simulink model "EMPlanner_cs"  (R2020a)
settings: Solver=ode5  StartTime=0.0  StopTime=120  FixedStep=1/1000  RelTol=1e-3
PreLoadFcn:
  | mbxruntime.callbacks.PreLoadFcn(bdroot);
PostLoadFcn:
  | mbxruntime.callbacks.PostLoadFcn(bdroot);
InitFcn:
  | mbxruntime.callbacks.InitFcn(bdroot);
StartFcn:
  | mbxruntime.callbacks.StartFcn(bdroot);
StopFcn:
  | mbxruntime.callbacks.StopFcn(bdroot);
model workspace (MAT data in the model file):
  mbox_table : object (value not decoded)
  model_closed = 0
  sim_status = 0
undefined symbols (not defined in the file or in its folder): aubr, c_factor, cf, cr, DiscIntNeverNeededParam, global_path_x, global_path_y, KD_PID_distance, KD_PID_speed, KI_PID_distance, KI_PID_speed, KP_PID_distance, KP_PID_speed, la, lb, LQR_K1, LQR_K2, LQR_K3, LQR_K4, m, rack_displacement, right_wheel_ground, tablebr, vubr, vx_break_point, warningInitialVelocity, x0
libraries: PreScanSimulinkLibrary x33, simulink x19, simulink_extras x6, Solver_SF x1
(part 6 of 11)

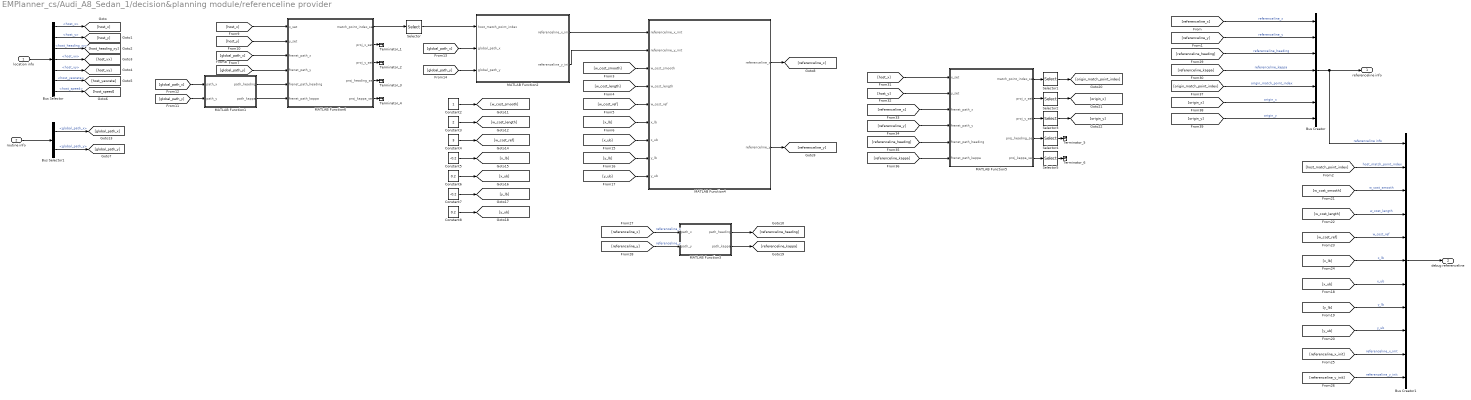
== system EMPlanner_cs/Audi_A8_Sedan_1/decision&planning module/referenceline provider ==
  location info : Inport
  routine info : Inport  Port=2
  Bus Creator : BusCreator  Inputs=7
  Bus Creator1 : BusCreator  Inputs=11
  Bus Selector : BusSelector  OutputSignals=host_x,host_y,host_heading_xy,host_vx,host_vy,host_yawrate,host_speed
  Bus Selector1 : BusSelector  OutputSignals=global_path_x,global_path_y
  Constant2 : Constant
  Constant3 : Constant  Value=2
  Constant4 : Constant  Value=3
  Constant5 : Constant  Value=-0.2
  Constant6 : Constant  Value=0.2
  Constant7 : Constant  Value=-0.2
  Constant8 : Constant  Value=0.2
  MATLAB Function1 : MATLAB Function  TreatAsAtomicUnit=on
  MATLAB Function2 : MATLAB Function  TreatAsAtomicUnit=on
  MATLAB Function3 : MATLAB Function  TreatAsAtomicUnit=on
  MATLAB Function4 : MATLAB Function  TreatAsAtomicUnit=on
  MATLAB Function5 : MATLAB Function  TreatAsAtomicUnit=on
  MATLAB Function6 : MATLAB Function  TreatAsAtomicUnit=on
  Selector{,1..5} (6 alike) : Selector  InputPortWidth=128  IndexOptions=Index vector (dialog)  Indices=1  OutputSizes=1
  Terminator_{1..6} (6 alike) : Terminator
  referenceline info : Outport
  debug referenceline : Outport  Port=2
  wires:
  [global_path_x] -> MATLAB Function2/2(global_path_x)
  [host_x] -> MATLAB Function6/1(x_set)
  MATLAB Function1/2(path_kappa) -> MATLAB Function6/6(frenet_path_kappa)
  MATLAB Function1/1(path_heading) -> MATLAB Function6/5(frenet_path_heading)
  [global_path_y] -> MATLAB Function6/4(frenet_path_y)
  [global_path_x] -> MATLAB Function6/3(frenet_path_x)
  [host_y] -> MATLAB Function6/2(y_set)
  [global_path_y] -> MATLAB Function1/2(path_y)
  [global_path_x] -> MATLAB Function1/1(path_x)
  Selector/1 -> MATLAB Function2/1(host_match_point_index)
  MATLAB Function6/1(match_point_index_set) -> Selector/1
  [global_path_y] -> MATLAB Function2/3(global_path_y)
  MATLAB Function2/1(referenceline_x_init) -> MATLAB Function4/1(referenceline_x_init)
  Bus Selector/5 -> [host_vy]  "<host_vy>"
  Bus Selector/1 -> [host_x]  "<host_x>"
  Bus Selector/2 -> [host_y]  "<host_y>"
  Bus Selector/3 -> [host_heading_xy]  "<host_heading_xy>"
  Bus Selector/4 -> [host_vx]  "<host_vx>"
  Bus Selector/7 -> [host_speed]  "<host_speed>"
  Bus Selector/6 -> [host_yawrate]  "<host_yawrate>"
  location info/1 -> Bus Selector/1
  Bus Selector1/2 -> [global_path_y]  "<global_path_y>"
  Bus Selector1/1 -> [global_path_x]  "<global_path_x>"
  routine info/1 -> Bus Selector1/1
  MATLAB Function4/1(referenceline_x) -> [referenceline_x]
  MATLAB Function4/2(referenceline_y) -> [referenceline_y]
  [referenceline_x] -> Bus Creator/1  "referenceline_x"
  [referenceline_y] -> Bus Creator/2  "referenceline_y"
  Bus Creator1/1 -> debug referenceline/1
  Bus Creator/1 -> Bus Creator1/1, referenceline info/1  "referenceline info"
  Constant2/1 -> [w_cost_smooth]
  Constant3/1 -> [w_cost_length]
  Constant8/1 -> [y_ub]
  Constant7/1 -> [y_lb]
  Constant6/1 -> [x_ub]
  Constant5/1 -> [x_lb]
  Constant4/1 -> [w_cost_ref]
  [w_cost_smooth] -> MATLAB Function4/3(w_cost_smooth)
  [w_cost_length] -> MATLAB Function4/4(w_cost_length)
  [w_cost_ref] -> MATLAB Function4/5(w_cost_ref)
  [x_lb] -> MATLAB Function4/6(x_lb)
  [x_ub] -> MATLAB Function4/7(x_ub)
  [y_lb] -> MATLAB Function4/8(y_lb)
  [y_ub] -> MATLAB Function4/9(y_ub)
  MATLAB Function2/2(referenceline_y_init) -> MATLAB Function4/2(referenceline_y_init)
  [w_cost_ref] -> Bus Creator1/5  "w_cost_ref"
  [x_lb] -> Bus Creator1/6  "x_lb"
  [w_cost_length] -> Bus Creator1/4  "w_cost_length"
  [x_ub] -> Bus Creator1/7  "x_ub"
  [w_cost_smooth] -> Bus Creator1/3  "w_cost_smooth"
  [y_lb] -> Bus Creator1/8  "y_lb"
  [host_match_point_index] -> Bus Creator1/2  "host_match_point_index"
  [y_ub] -> Bus Creator1/9  "y_ub"
  [referenceline_x_init] -> Bus Creator1/10  "referenceline_x_init"
  [referenceline_y_init] -> Bus Creator1/11  "referenceline_y_init"
  [referenceline_x] -> MATLAB Function3/1(path_x)  "referenceline_x"
  [referenceline_y] -> MATLAB Function3/2(path_y)  "referenceline_y"
  MATLAB Function3/1(path_heading) -> [referenceline_heading]
  MATLAB Function3/2(path_kappa) -> [referenceline_kappa]
  [referenceline_kappa] -> Bus Creator/4  "referenceline_kappa"
  [referenceline_heading] -> Bus Creator/3  "referenceline_heading"
  [host_x] -> MATLAB Function5/1(x_set)
  [host_y] -> MATLAB Function5/2(y_set)
  [referenceline_x] -> MATLAB Function5/3(frenet_path_x)
  [referenceline_y] -> MATLAB Function5/4(frenet_path_y)
  [referenceline_heading] -> MATLAB Function5/5(frenet_path_heading)
  [referenceline_kappa] -> MATLAB Function5/6(frenet_path_kappa)
  MATLAB Function5/1(match_point_index_set) -> Selector1/1
  MATLAB Function5/2(proj_x_set) -> Selector2/1
  MATLAB Function5/3(proj_y_set) -> Selector3/1
  MATLAB Function5/4(proj_heading_set) -> Selector4/1
  MATLAB Function5/5(proj_kappa_set) -> Selector5/1
  Selector1/1 -> [origin_match_point_index]
  Selector2/1 -> [origin_x]
  Selector3/1 -> [origin_y]
  [origin_match_point_index] -> Bus Creator/5  "origin_match_point_index"
  [origin_x] -> Bus Creator/6  "origin_x"
  [origin_y] -> Bus Creator/7  "origin_y"
  MATLAB Function6/2(proj_x_set) -> Terminator_1/1
  MATLAB Function6/3(proj_y_set) -> Terminator_2/1
  MATLAB Function6/4(proj_heading_set) -> Terminator_3/1
  MATLAB Function6/5(proj_kappa_set) -> Terminator_4/1
  Selector4/1 -> Terminator_5/1
  Selector5/1 -> Terminator_6/1

== system EMPlanner_cs/Audi_A8_Sedan_2/Dynamics_Simple/Chassis ==
  TransmissionTorque_[Nm] : Inport
  BrakePressure_[bar] : Inport  Port=2
  DeltaSteer_[deg] : Inport  Port=3
  Initial_Vx_[m s-1] : Inport  Port=4
  Abs : Abs
  Bicycle_model_[XYZ] : Subsystem
      mask Display: image(imread('Bicycle_model.png'));
  Constant3 : Constant  Value=[0 0]
  Constant4 : Constant  Value=[0 0]
  Degrees to Radians : simulink_extras/Transformations/Degrees to Radians
  FinalDriveRatio : Gain  Gain=p.Rfd  SaturateOnIntegerOverflow=on  OutDataTypeStr=Inherit: Same as input  ParamDataTypeStr=Inherit: Same as input
  "FinalDriveRatio " : Gain  Gain=p.Rfd  SaturateOnIntegerOverflow=on  OutDataTypeStr=Inherit: Same as input  ParamDataTypeStr=Inherit: Same as input
  FrontTyre : Subsystem
      mask Display: image(imread('Tyre.png'));
  Gain : Gain  Gain=2*pi/60
  MuxDynState : Subsystem
  Power Assisted Steering : Subsystem
  Product : Product  RndMeth=Zero
  RearTyre : Subsystem
      mask Display: image(imread('Tyre.png'));
  SteerRatio : Gain  Gain=1/p.SteerRatio
  Terminator4 : Terminator
  "[ms-1 --> rpm]" : Gain  Gain=60/(2*pi*p.Rw)  SaturateOnIntegerOverflow=on  OutDataTypeStr=Inherit: Same as input  ParamDataTypeStr=Inherit: Same as input
  to_kW : Gain  Gain=0.001
  State : Outport
  VehicleSpeed_[ms-1] : Outport  Port=2
  Vy_[ms-1] : Outport  Port=3
  ax_[ms-2] : Outport  Port=4
  ay_[ms-2] : Outport  Port=5
  PDrive_[kW] : Outport  Port=6
  TransmissionOut_[rpm] : Outport  Port=7
  wires:
  [vy] -> Vy_[ms-1]/1  "vy_[ms-1]"
  to_kW/1 -> PDrive_[kW]/1  "PDrive_[kW]"
  Gain/1 -> Product/1
  Bicycle_model_[XYZ]/10(ax_[ms-2]) -> ax_[ms-2]/1  "ax_[ms-2]"
  Product/1 -> to_kW/1
  [DT] -> Product/2
  Bicycle_model_[XYZ]/11(ay_[ms-2]) -> ay_[ms-2]/1  "ay_[ms-2]"
  Abs/1 -> Bicycle_model_[XYZ]/7(|vx|_[ms-1])
  Degrees to Radians/1 -> SteerRatio/1
  [vx] -> Abs/1
  SteerRatio/1 -> [DeltaWheel], Bicycle_model_[XYZ]/1(DeltaWheel_[rad])  "DeltaWheel_[rad]"
  TransmissionTorque_[Nm]/1 -> "FinalDriveRatio "/1  "DriveTorque_[Nm]"
  RearTyre/1(FyRear_[N]) -> Bicycle_model_[XYZ]/8(Fy_rear_[N])  "Fy_rear_[N]"
  FrontTyre/1(FyFront_[N]) -> Bicycle_model_[XYZ]/9(Fy_front_[N])  "Fy_front_[N]"
  Bicycle_model_[XYZ]/1(|vx|_[ms-1]1) -> [Absvx]  "|vx|_[ms-1]"
  Bicycle_model_[XYZ]/2(vy_[ms-1]) -> [vy], MuxDynState/2(vy [ms-1])  "Vy_[ms-1]"
  Bicycle_model_[XYZ]/4(RollAngle_[rad]) -> MuxDynState/4(R [rad]), [RollAngle]  "RollAngle_[rad]"
  Bicycle_model_[XYZ]/6(YawAngle_[rads-1]) -> [YawRate]  "YawRate_[rad s-1]"
  Bicycle_model_[XYZ]/7(Vx_[ms-1]) -> [vx]  "Vx_[ms-1]"
  [DeltaWheel] -> FrontTyre/1(DeltaWheel_[rad])
  [Absvx] -> FrontTyre/2(|vx|_[ms-1])
  [vy] -> FrontTyre/3(vy_[ms-1])
  [YawRate] -> FrontTyre/4(dYawAngle_[rads-1])
  [Absvx] -> RearTyre/1(|vx|_[ms-1])
  [vy] -> RearTyre/2(vy_[ms-1])
  [YawRate] -> RearTyre/3(dpsi_[rads-1])
  Bicycle_model_[XYZ]/3(vz_[ms-1]) -> MuxDynState/3(vz [ms-1])  "Vz_[ms-1]"
  Bicycle_model_[XYZ]/8(PitchAngle_[rad]) -> MuxDynState/5(P [rad])  "PitchAngle_[rad]"
  Bicycle_model_[XYZ]/9(YawAngle_[rad]) -> MuxDynState/6(Y [rad])  "YawAngle_[rad]"
  "[ms-1 --> rpm]"/1 -> Gain/1, FinalDriveRatio/1
  FinalDriveRatio/1 -> TransmissionOut_[rpm]/1  "TransmissionOut_[rpm]"
  [vx] -> "[ms-1 --> rpm]"/1, VehicleSpeed_[ms-1]/1, MuxDynState/1(vx [ms-1])  "vx_[ms-1]"
  [vx] -> Power Assisted Steering/1(Vx_[ms-1])
  DeltaSteer_[deg]/1 -> Power Assisted Steering/2(Delta_in_[deg])
  Power Assisted Steering/1(Delta_out_[deg]) -> Degrees to Radians/1
  [RollAngle] -> FrontTyre/5(RollAngle_[rad])
  [RollAngle] -> RearTyre/4(RollAngle_[rad])
  Constant3/1 -> Bicycle_model_[XYZ]/2(zFront_[m]_dzFront_[ms-1])  "zFront_[m]_dzFront_[m s-1]"
  Constant4/1 -> Bicycle_model_[XYZ]/3(zRear_[m]_dzRear_[ms-1])  "zRear_[m]_dzRear_[m s-1]"
  BrakePressure_[bar]/1 -> Bicycle_model_[XYZ]/4(BrakePressure_[bar])  "BrakePressure_[bar]"
  "FinalDriveRatio "/1 -> Bicycle_model_[XYZ]/5(DriveTorque_[Nm]), [DT]  "DriveTorque_[Nm]"
  Initial_Vx_[m s-1]/1 -> Bicycle_model_[XYZ]/6(v0_[ms-1])  "Initial_Vx_[m s-1]"
  Bicycle_model_[XYZ]/5(RollRate_[rads-1]) -> Terminator4/1  "RollRate_[rad s-1]"
  MuxDynState/1(State) -> State/1  "State"

== system EMPlanner_cs/Audi_A8_Sedan_2/Dynamics_Simple/Engine ==
  ImpellerTorque_[Nm] : Inport
  Throttle_[%] : Inport  Port=2
  Configurable Subsystem : Subsystem  BlockChoice=Rate Limiter  mask{ComputationMode=ComputationMode}
      mask prompts: ComputationMode "Compuation mode:"
      mask init:
      | SetComputationMode(gcb,ComputationMode);
      settings: AttributesFormatString=%<BlockChoice>  OpenFcn=BringToFront(gcb);  MemberBlocks=Discrete Rate Limiter,Rate Limiter
      settings: TemplateBlock=|
      | PreScanSimulinkLibrary/Configurable Subsystems/TransferFunction
      | Engine/Configurable
      | Subsystem
  Configurable Subsystem1 : Subsystem  BlockChoice=Integrator  mask{ComputationMode=ComputationMode}
      mask prompts: ComputationMode "Computation mode:"
      mask init:
      | SetComputationMode(gcb,ComputationMode);
      settings: AttributesFormatString=%<BlockChoice>  OpenFcn=BringToFront(gcb);  MemberBlocks=Discrete-Time Integrator,Integrator
      settings: TemplateBlock=|
      | PreScanSimulinkLibrary/Configurable Subsystems/integral with initial condition and limts
      | for engine/Configurable
      | Subsystem
  EngineTorque : Lookup2D  RowIndex=p.thvec  ColumnIndex=p.nevec  Table=p.emap  InputSameDT=on
  Gain : Gain  Gain=2*pi/60
  Product : Product  RndMeth=Zero
  Sum : Sum  Inputs=-+  InputSameDT=on  SaturateOnIntegerOverflow=on  OutDataTypeStr=Inherit: Same as first input
  engine + impeller inertia : Gain  Gain=1/p.Iei  SaturateOnIntegerOverflow=on  OutDataTypeStr=Inherit: Same as input  ParamDataTypeStr=Inherit: Same as input
  rad|sec2rpm : Gain  Gain=60/2/pi  SaturateOnIntegerOverflow=on  OutDataTypeStr=Inherit: Same as input  ParamDataTypeStr=Inherit: Same as input
  to_kW : Gain  Gain=0.001
  nEngine_[rpm] : Outport  InitialOutput=0
  PEngine_[kW] : Outport  Port=2  InitialOutput=0
  wires:
  rad|sec2rpm/1 -> nEngine_[rpm]/1, EngineTorque/2, Gain/1  "rpm"
  engine + impeller inertia/1 -> Configurable Subsystem1/1(In1)  "rads-2"
  EngineTorque/1 -> Sum/2, Product/2
  Sum/1 -> engine + impeller inertia/1
  Configurable Subsystem1/1(Out1) -> rad|sec2rpm/1  "rads-1"
  Throttle_[%]/1 -> Configurable Subsystem/1(In1)
  ImpellerTorque_[Nm]/1 -> Sum/1
  Configurable Subsystem/1(Out1) -> EngineTorque/1
  Product/1 -> to_kW/1
  Gain/1 -> Product/1
  to_kW/1 -> PEngine_[kW]/1

== system EMPlanner_cs/Audi_A8_Sedan_2/Dynamics_Simple/Gear: Auto Manual ==
  note: 0; Auto = on // Manual =off
      | 1; Auto = off // Manual =on
  Auto_Manual : Inport
  Manual_Gear : Inport  Port=2
  Auto_Gear : Inport  Port=3
  If : If  IfExpression=u1 == 0
  If Action Subsystem : Subsystem  TreatAsAtomicUnit=on
  If Action Subsystem1 : Subsystem  TreatAsAtomicUnit=on
  Merge : Merge
  Gear : Outport
  wires:
  If Action Subsystem/1(Out1) -> Merge/1
  Auto_Gear/1 -> If Action Subsystem/1(In1)
  If/1 -> If Action Subsystem/Action
  Merge/1 -> Gear/1
  If Action Subsystem1/1(Out1) -> Merge/2
  Manual_Gear/1 -> If Action Subsystem1/1(In1)
  If/2 -> If Action Subsystem1/Action
  Auto_Manual/1 -> If/1

== system EMPlanner_cs/Audi_A8_Sedan_2/Dynamics_Simple/ShiftLogic ==
  Throttle_[%] : Inport
  GearNr_[-] : Inport  Port=2
  Auto_GearShift : Inport  Port=3
  VehSpeed_[ms-1] : Inport  Port=4
  Add2 : Sum
  Data Type Conversion1 : DataTypeConversion  OutDataTypeStr=double
  Detect Increase1 : simulink/Logic and Bit Operations/Detect Increase  vinit=0.0  OutDataTypeStr=uint8
  Detect Increase : Subsystem
  Gear limitation : Saturate  UpperLimit=p.maxGear  LowerLimit=1
  Gear limitation while shifting : Saturate  UpperLimit=p.maxGear  LowerLimit=1
  GearNeutral : Constant  Value=0
  GearReverse : Constant  Value=-1
  "IC, gear = 1" : Memory  InitialCondition=1  InheritSampleTime=on
  If Action Neutral : Subsystem  TreatAsAtomicUnit=on
  If Action Normal : Subsystem  TreatAsAtomicUnit=on
  If Action Reverse : Subsystem  TreatAsAtomicUnit=on
  Memory : Memory  InheritSampleTime=on
  Merge : Merge  Inputs=3
  Relational Operator : RelationalOperator  OutDataTypeStr=boolean  RndMeth=Nearest
  Relational Operator1 : RelationalOperator  Operator=<=  OutDataTypeStr=boolean  RndMeth=Nearest
  Shift_Down time : Delay  DelayLength=p.ShiftDown_fac
  Shift_Up time : Delay  DelayLength=p.ShiftUp_fac
  Sum : Sum  Inputs=+-
  interp_down : Lookup2D  RowIndex=p.downth  ColumnIndex=[1:p.maxGear]  Table=p.downtab  LookUpMeth=Interpolation-Use End Values  InputSameDT=on
  interp_up : Lookup2D  RowIndex=p.upth  ColumnIndex=[1:p.maxGear]  Table=p.uptab  LookUpMeth=Interpolation-Use End Values  InputSameDT=on
  reverse/neutral/normal gear : If  IfExpression=u1 == 0  ElseIfExpressions=u1 < 0
  to_ms-1 : Gain  Gain=1/3.6
  "to_ms-1 " : Gain  Gain=1/3.6
  GearNr : Outport
  wires:
  Auto_GearShift/1 -> reverse/neutral/normal gear/1
  "IC, gear = 1"/1 -> If Action Normal/1(In1)
  Merge/1 -> GearNr/1
  If Action Reverse/1(Out1) -> Merge/2
  If Action Neutral/1(Out1) -> Merge/1
  If Action Normal/1(Out1) -> Merge/3
  reverse/neutral/normal gear/3 -> If Action Normal/Action
  reverse/neutral/normal gear/1 -> If Action Neutral/Action
  reverse/neutral/normal gear/2 -> If Action Reverse/Action
  GearReverse/1 -> If Action Reverse/1(In1)
  GearNeutral/1 -> If Action Neutral/1(In1)
  Shift_Down time/1 -> Sum/2
  Shift_Up time/1 -> Sum/1
  Detect Increase/1(Out1) -> Shift_Up time/1
  Data Type Conversion1/1 -> Shift_Down time/1
  Detect Increase1/1 -> Data Type Conversion1/1
  Sum/1 -> Add2/1
  Memory/1 -> Add2/2  "GearNr_[-]"
  Add2/1 -> Gear limitation while shifting/1
  Gear limitation while shifting/1 -> "IC, gear = 1"/1, Memory/1  "GearNr_[-]"
  Throttle_[%]/1 -> interp_down/1, interp_up/1
  Relational Operator/1 -> Detect Increase/2(In2)
  Relational Operator1/1 -> Detect Increase1/1
  interp_down/1 -> "to_ms-1 "/1
  VehSpeed_[ms-1]/1 -> Relational Operator/1, Relational Operator1/1
  interp_up/1 -> to_ms-1/1
  Gear limitation/1 -> interp_down/2, interp_up/2, Detect Increase/1(GearNr_[-])
  GearNr_[-]/1 -> Gear limitation/1
  to_ms-1/1 -> Relational Operator/2
  "to_ms-1 "/1 -> Relational Operator1/2

== system EMPlanner_cs/Audi_A8_Sedan_2/Dynamics_Simple/Transmission ==
  nEngine_[rpm] : Inport
  GearNr_[-] : Inport  Port=2
  n_TransmissionOut_[rpm] : Inport  Port=3
  Torque_Converter : Subsystem
      mask Display: image(imread('TorqueConverter.png'));
  Transmission_Ratio : Subsystem
  Viscous coupling : Lookup  InputValues=[-5:0.1:5]*p.m/4  Table=p.m/4*tanh([-5:0.1:5])
  ImpellerTorque_[Nm] : Outport  InitialOutput=0
  TransmissionTorque_[Nm] : Outport  Port=2  InitialOutput=0
  wires:
  Torque_Converter/2(TurbineTorque_[Nm]) -> Viscous coupling/1  "Converter_Torque_[Nm]"
  Transmission_Ratio/2(nTransmissionIn_[rpm]) -> Torque_Converter/2(nTransmission_[rpm])
  nEngine_[rpm]/1 -> Torque_Converter/1(nEngine_[rpm])
  GearNr_[-]/1 -> Transmission_Ratio/2(GearNr_[-]), Torque_Converter/3(Gear nr)
  n_TransmissionOut_[rpm]/1 -> Transmission_Ratio/3(nTransmissionOut_[rpm])
  Torque_Converter/1(ImpellerTorque_[Nm]) -> ImpellerTorque_[Nm]/1
  Transmission_Ratio/1(tTransmissionOut_[Nm]) -> TransmissionTorque_[Nm]/1
  Viscous coupling/1 -> Transmission_Ratio/1(tTransmissionIn_[Nm])

== system EMPlanner_cs/Audi_A8_Sedan_2/PathFollower_Preview_1/LateralController ==
  TrajOffset x,y,Y [m,m,deg] : Inport
  ActorOffset_Left(+) / Right(-) [m] : Inport  Port=2
  position x,y,Y [m,m,deg] : Inport  Port=3
  vx [m/s] : Inport  Port=4
  vy [m/s] : Inport  Port=5
  Yaw rate [deg/s] : Inport  Port=6
  CorneringStiffness_Tyres_Front [N/rad] : Inport  Port=7
  CorneringStiffness_Tyres_Rear [N/rad] : Inport  Port=8
  steering_ratio[-] : Inport  Port=9
  Avoid_0 : Saturate  UpperLimit=1000  LowerLimit=0.1
  CTRL REFERENCES : Subsystem
  Calculate delta steering error : Subsystem
      mask Display:
      | port_label('input', 1, 'v_x_vehicle [m/s]')
      | port_label('input', 2, 'v_x_vehicle_Min [m/s]')
      | port_label('input', 3, 't_Preview_LatCtrl [s]')
      | port_label('input', 4, 'v_y_vehicle [m/s]')
      | port_label('input', 5, 'yawrate_vehicle [rad/sec]')
      | port_label('input', 6, 'CorneringStiffness_Tyres_Front [N/rad]')
      | port_label('input', 7, 'CorneringStiffness_Tyres_Rear [N/rad]')
      | port_label('input', 8, 'm_vehicle_total [kg]')
      | port_label('input', 9, 'inertia_z_vehicle_total [kg m2]')
      | port_label('input', 10, 'e_Lat [m]')
      | port_label('input', 11, 'Distance_frontaxle_COG(+) [m]')
      | port_label('input', 12, 'wheel_base [m]')
      | port_label('output', 1, 'delta_steeringwheel [rad]')
  Const_t_Preview_LatCtrl[s] : Constant  Value=PreviewTime  SampleTime=CSSampleTime
  Const_v_x_Vehicle_Min[km|h] : Constant  Value=LowSpeedLimit  SampleTime=CSSampleTime
  Constant6 : Constant  SampleTime=CSSampleTime
  Demux : Demux  Outputs=3
  Demux1 : Demux  Outputs=3
  Distance_frontaxle_COG(+) [m] : Constant  Value=length_a  SampleTime=CSSampleTime
  Gain : Gain  Gain=1*pi/180
  Gain1 : Gain  Gain=1*pi/180
  Gain4 : Gain
  Memory : Memory  InheritSampleTime=on
  Memory1 : Memory  InheritSampleTime=on
  Memory2 : Memory  InheritSampleTime=on
  Mux : Mux  Inputs=3
  Mux1 : Mux  Inputs=3
  SteeringWheelAngle : Subsystem
  deg to rad : Gain  Gain=pi/180
  inertia_z_vehicle_total [kg m2] : Constant  Value=Jzz  SampleTime=CSSampleTime
  km|h to m|s : Gain  Gain=1/3.6
  m_vehicle_total_[kg] : Constant  Value=mass  SampleTime=CSSampleTime
  s_Preview_LatCtrl : Subsystem
  wheel_base [m] : Constant  Value=length_l  SampleTime=CSSampleTime
  Actor/Traj_distance [m] : Outport
  Actor/Traj_angle [deg] : Outport  Port=2
  delta_steerwheel [deg] : Outport  Port=3
  wires:
  km|h to m|s/1 -> Calculate delta steering error/2(In2), s_Preview_LatCtrl/2(v_x_Vehicle_Min[m|s])
  Gain/1 -> Mux/3
  Mux/1 -> CTRL REFERENCES/3(TrajOffset [m,m,rad])
  ActorOffset_Left(+) / Right(-) [m]/1 -> CTRL REFERENCES/4(ActorOffset_Left(+) / Right(-)_[m])
  Demux/1 -> Mux/1
  Demux/2 -> Mux/2
  Demux/3 -> Gain/1
  TrajOffset x,y,Y [m,m,deg]/1 -> Demux/1
  CTRL REFERENCES/2(Actor/Traj_angle [deg]) -> Actor/Traj_angle [deg]/1
  CTRL REFERENCES/1(Actor/Traj_distance [m]) -> Actor/Traj_distance [m]/1
  Calculate delta steering error/1(Out1) -> SteeringWheelAngle/1(Angle_Steering[rad])
  vx [m/s]/1 -> Memory1/1
  vy [m/s]/1 -> Memory2/1
  CorneringStiffness_Tyres_Front [N/rad]/1 -> Calculate delta steering error/6(In6)
  m_vehicle_total_[kg]/1 -> Calculate delta steering error/8(In8)
  inertia_z_vehicle_total [kg m2]/1 -> Calculate delta steering error/9(In9)
  steering_ratio[-]/1 -> SteeringWheelAngle/2(i_Steering[])
  SteeringWheelAngle/1(Angle_SteeringWheel[deg]) -> Gain4/1, Memory/1
  Memory/1 -> SteeringWheelAngle/3(Angle_SteeringWheel_Last[deg])
  Constant6/1 -> SteeringWheelAngle/4(LatCtrl1_Enable[0Off|1On])
  Avoid_0/1 -> Calculate delta steering error/3(In3), s_Preview_LatCtrl/3(t_Preview_LatCtrl[s])
  Const_v_x_Vehicle_Min[km|h]/1 -> km|h to m|s/1
  s_Preview_LatCtrl/1(s_Preview_LatCtrl[m]) -> CTRL REFERENCES/2(Position Preview Distance [m])
  Const_t_Preview_LatCtrl[s]/1 -> Avoid_0/1
  Gain4/1 -> delta_steerwheel [deg]/1
  Distance_frontaxle_COG(+) [m]/1 -> Calculate delta steering error/11(In11)
  CorneringStiffness_Tyres_Rear [N/rad]/1 -> Calculate delta steering error/7(In7)
  Yaw rate [deg/s]/1 -> deg to rad/1
  deg to rad/1 -> Calculate delta steering error/5(In5)
  Gain1/1 -> Mux1/3
  Demux1/1 -> Mux1/1
  Demux1/2 -> Mux1/2
  Demux1/3 -> Gain1/1
  position x,y,Y [m,m,deg]/1 -> Demux1/1
  Mux1/1 -> CTRL REFERENCES/1(Pos x,y,Y [m,m,rad])
  wheel_base [m]/1 -> Calculate delta steering error/12(In12)
  CTRL REFERENCES/3(e_Lat [m]) -> Calculate delta steering error/10(In10)
  Memory1/1 -> Calculate delta steering error/1(In1), s_Preview_LatCtrl/1(v_x_Vehicle[m|s])
  Memory2/1 -> Calculate delta steering error/4(In4)

== system EMPlanner_cs/Audi_A8_Sedan_2/PathFollower_Preview_1/LongitudinalController ==
  v_actual [m/s] : Inport
  Desired Velocity [m/s] : Inport  Port=2
  Initial Velocity [m/s] : Inport  Port=3
  Check_Initial_Velocity : Subsystem
  Demux : Demux  Outputs=3
  GearNormal : Constant
  "GearNormal " : Constant
  If Desired Velocity = 0 : Subsystem  TreatAsAtomicUnit=on
  If Desired Velocity ~= 0 : Subsystem  TreatAsAtomicUnit=on
  Memory External IC : Subsystem
  Merge : Merge
  Mux : Mux  Inputs=3
  Mux2 : Mux  Inputs=3
  Sum4 : Sum  Inputs=|+-
  if : If  IfExpression=u1 == 0  SampleTime=CSSampleTime
  throttle [%] : Outport
  brake pressure [bar] : Outport  Port=2
  v0 [m/s] : Outport  Port=3
  Auto_GearShift : Outport  Port=4
  wires:
  v_actual [m/s]/1 -> Check_Initial_Velocity/1(" v_actual_[m|s]"), Memory External IC/1(u)
  Memory External IC/1(y) -> Sum4/2
  Sum4/1 -> If Desired Velocity ~= 0/2(Desired Velocity [m/s])
  Desired Velocity [m/s]/1 -> if/1, Sum4/1
  Initial Velocity [m/s]/1 -> Check_Initial_Velocity/2(Initial_Velocity_[m|s]), Memory External IC/2(IC), v0 [m/s]/1
  GearNormal/1 -> If Desired Velocity = 0/1(In1)
  Merge/1 -> Demux/1
  If Desired Velocity = 0/1(throttle [%]) -> Mux/1
  If Desired Velocity = 0/2(brake pressure [bar]) -> Mux/2
  Mux2/1 -> Merge/2
  Mux/1 -> Merge/1
  Demux/1 -> throttle [%]/1
  Demux/2 -> brake pressure [bar]/1
  Demux/3 -> Auto_GearShift/1
  "GearNormal "/1 -> If Desired Velocity ~= 0/1(In1)
  If Desired Velocity = 0/3(Auto_GearShift) -> Mux/3
  if/2 -> If Desired Velocity ~= 0/Action
  if/1 -> If Desired Velocity = 0/Action
  If Desired Velocity ~= 0/1(throttle [%]) -> Mux2/1
  If Desired Velocity ~= 0/2(brake pressure [bar]) -> Mux2/2
  If Desired Velocity ~= 0/3(Auto_GearShift) -> Mux2/3

== system EMPlanner_cs/Audi_A8_Sedan_2/SELF_Demux/compas converter ==
  rotz [rad] : Inport
  cart2compas : Subsystem
  rad2deg : Gain  Gain=180/pi
  heading [deg] : Outport
  wires:
  rad2deg/1 -> cart2compas/1(Angle [deg])
  rotz [rad]/1 -> rad2deg/1
  cart2compas/1(heading [deg]) -> heading [deg]/1

== system EMPlanner_cs/Audi_A8_Sedan_2/Trajectories/Traj2State1 ==
  Traj Org : Inport
  Offset : Inport  Port=2
  Add2 : Sum
  ApplyRotation : PreScanSimulinkLibrary/ApplyRotation  SystemSampleTime=-1  Latency=0  AutoFrameSizeCalculation=off
  ApplyRotation1 : PreScanSimulinkLibrary/ApplyRotation  SystemSampleTime=-1  Latency=0  AutoFrameSizeCalculation=off
  ApplyRotation2 : PreScanSimulinkLibrary/ApplyRotation  SystemSampleTime=-1  Latency=0  AutoFrameSizeCalculation=off
  Constant : Constant  Value=zeros(12,1)
  Mux : Mux  Inputs=6
  Mux1 : Mux  Inputs=2
  Mux{2,4..9} (7 alike) : Mux  Inputs=3
  Mux3 : Mux  Inputs=2
  Selector : Selector  InputPortWidth=6  IndexOptions=Index vector (dialog)  Indices=[4 5 6]  OutputSizes=1
  Selector1 : Selector  InputPortWidth=21  IndexOptions=Index vector (dialog)  Indices=[5]  OutputSizes=1
  Selector10 : Selector  InputPortWidth=21  IndexOptions=Index vector (dialog)  Indices=[2]  OutputSizes=1
  Selector11 : Selector  InputPortWidth=21  IndexOptions=Index vector (dialog)  Indices=[3]  OutputSizes=1
  Selector12 : Selector  InputPortWidth=21  IndexOptions=Index vector (dialog)  Indices=[1]  OutputSizes=1
  Selector13 : Selector  InputPortWidth=21  IndexOptions=Index vector (dialog)  Indices=[8]  OutputSizes=1
  Selector14 : Selector  InputPortWidth=21  IndexOptions=Index vector (dialog)  Indices=[9]  OutputSizes=1
  Selector15 : Selector  InputPortWidth=21  IndexOptions=Index vector (dialog)  Indices=[7]  OutputSizes=1
  Selector16 : Selector  InputPortWidth=21  IndexOptions=Index vector (dialog)  Indices=[14]  OutputSizes=1
  Selector17 : Selector  InputPortWidth=21  IndexOptions=Index vector (dialog)  Indices=[15]  OutputSizes=1
  Selector18 : Selector  InputPortWidth=21  IndexOptions=Index vector (dialog)  Indices=[13]  OutputSizes=1
  Selector19 : Selector  InputPortWidth=21  IndexOptions=Index vector (dialog)  Indices=[20]  OutputSizes=1
  Selector2 : Selector  InputPortWidth=21  IndexOptions=Index vector (dialog)  Indices=[6]  OutputSizes=1
  Selector20 : Selector  InputPortWidth=21  IndexOptions=Index vector (dialog)  Indices=[21]  OutputSizes=1
  Selector21 : Selector  InputPortWidth=21  IndexOptions=Index vector (dialog)  Indices=[19]  OutputSizes=1
  Selector3 : Selector  InputPortWidth=21  IndexOptions=Index vector (dialog)  Indices=[12]  OutputSizes=1
  Selector4 : Selector  InputPortWidth=21  IndexOptions=Index vector (dialog)  Indices=[17]  OutputSizes=1
  Selector5 : Selector  InputPortWidth=21  IndexOptions=Index vector (dialog)  Indices=[18]  OutputSizes=1
  Selector6 : Selector  InputPortWidth=21  IndexOptions=Index vector (dialog)  Indices=[16]  OutputSizes=1
  Selector7 : Selector  InputPortWidth=21  IndexOptions=Index vector (dialog)  Indices=[11]  OutputSizes=1
  Selector8 : Selector  InputPortWidth=21  IndexOptions=Index vector (dialog)  Indices=[10]  OutputSizes=1
  Selector9 : Selector  InputPortWidth=21  IndexOptions=Index vector (dialog)  Indices=[4]  OutputSizes=1
  Traj2State2 : Subsystem
  state : Outport
  wires:
  Mux9/1 -> ApplyRotation2/2, ApplyRotation1/2, ApplyRotation/2
  Selector20/1 -> Mux9/3
  Selector19/1 -> Mux9/2
  Selector21/1 -> Mux9/1
  Selector5/1 -> Mux8/3
  Selector4/1 -> Mux8/2
  Selector6/1 -> Mux8/1
  Mux8/1 -> Mux/6
  Mux6/1 -> ApplyRotation2/1
  Mux7/1 -> Mux/4
  ApplyRotation2/1 -> Mux/5
  Selector3/1 -> Mux7/3
  Selector7/1 -> Mux7/2
  Selector8/1 -> Mux7/1
  Mux4/1 -> Mux/2
  Mux5/1 -> ApplyRotation1/1
  ApplyRotation1/1 -> Mux/3
  Mux2/1 -> ApplyRotation/1
  ApplyRotation/1 -> Mux/1
  Selector2/1 -> Mux4/3
  Selector1/1 -> Mux4/2
  Selector9/1 -> Mux4/1
  Selector17/1 -> Mux6/3
  Selector16/1 -> Mux6/2
  Selector18/1 -> Mux6/1
  Selector14/1 -> Mux5/3
  Selector13/1 -> Mux5/2
  Selector15/1 -> Mux5/1
  Selector11/1 -> Mux2/3
  Selector10/1 -> Mux2/2
  Selector12/1 -> Mux2/1
  Mux3/1 -> Selector8/1, Selector7/1, Selector3/1, Selector18/1, Selector16/1, Selector17/1, Selector6/1, Selector20/1, Selector19/1, Selector21/1, Selector5/1, Selector4/1, Selector14/1, Selector13/1, Selector15/1, Selector2/1, Selector1/1, Selector9/1, Selector12/1, Selector10/1, Selector11/1
  Mux1/1 -> Add2/2
  Constant/1 -> Mux1/2
  Add2/1 -> Traj2State2/1(traj)
  Selector/1 -> Mux3/2
  Traj Org/1 -> Mux3/1
  Offset/1 -> Mux1/1, Selector/1
  Mux/1 -> Add2/1
  Traj2State2/1(state) -> state/1

== system EMPlanner_cs/Audi_A8_Sedan_2/Trajectories/TrajCoGOffset ==
  State In : Inport
  Add : Sum  Inputs=+-+
  Add1 : Sum
  ApplyRotation : PreScanSimulinkLibrary/ApplyRotation  SystemSampleTime=-1  Latency=0  AutoFrameSizeCalculation=off
  ApplyRotation1 : PreScanSimulinkLibrary/ApplyRotation  SystemSampleTime=-1  Latency=0  AutoFrameSizeCalculation=off
  CoG Offset : Constant  Value=[0 0 CoGOffsetZ]
  Degrees to Radians : simulink_extras/Transformations/Degrees to Radians
  Demux1 : Demux  Outputs=[3 3 3]
  Mux : Mux  Inputs=[3 3 3]
  Orientation : Constant  Value=[InitRoll InitPitch 0]
  State Out : Outport
  wires:
  State In/1 -> Demux1/1
  Demux1/1 -> Add/1
  Add/1 -> Mux/1
  Demux1/3 -> Mux/3, Add1/2
  Mux/1 -> State Out/1
  Demux1/2 -> Mux/2
  Orientation/1 -> Degrees to Radians/1
  ApplyRotation/1 -> Add/3
  ApplyRotation1/1 -> Add/2
  Add1/1 -> ApplyRotation/2
  CoG Offset/1 -> ApplyRotation1/1, ApplyRotation/1
  Degrees to Radians/1 -> Add1/1, ApplyRotation1/2

== system EMPlanner_cs/Audi_A8_Sedan_2/Trajectories/Trajectory_1 ==
  From Workspace : FromWorkspace  VariableName=trajectory  SampleTime=TimeStep  ZeroCross=off  OutputAfterFinalValue=Holding final value
  From Workspace1 : FromWorkspace  VariableName=trajectory  SampleTime=TimeStep  ZeroCross=off  OutputAfterFinalValue=Setting to zero
  Mux : Mux  Inputs=2
  Selector1 : Selector  InputPortWidth=24  IndexOptions=Index vector (dialog)  Indices=[7:18]  OutputSizes=1
  Selector9 : Selector  InputPortWidth=24  IndexOptions=Index vector (dialog)  Indices=[1:6]  OutputSizes=1
  trajectory : Outport
  wires:
  From Workspace/1 -> Selector9/1
  From Workspace1/1 -> Selector1/1
  Mux/1 -> trajectory/1
  Selector9/1 -> Mux/1
  Selector1/1 -> Mux/2

== system EMPlanner_cs/Box_1/Dynamics_Empty/MuxState ==
  note: mode: Dynamics
  note: mode: Positioning
  note: mode: Dynamics
      | VelVEHICLE
      | wrt VEH
  note: AnglesVEHICLE
      | wrtGLOB
  note: For state mode 'Dynamic' positions
      | are not taken into account, as they
      | are computed by integrating velocity.
      | Click annotation for Help.
  x [m] : Inport  SampleTime=TimeStep
  y [m] : Inport  Port=2  SampleTime=TimeStep
  z [m] : Inport  Port=3  SampleTime=TimeStep
  dx [m/s] : Inport  Port=4  SampleTime=TimeStep
  dy [m/s] : Inport  Port=5  SampleTime=TimeStep
  dz [m/s] : Inport  Port=6  SampleTime=TimeStep
  R [rad] : Inport  Port=7  SampleTime=TimeStep
  P [rad] : Inport  Port=8  SampleTime=TimeStep
  Y [rad] : Inport  Port=9  SampleTime=TimeStep
  Constant : Constant  DisableCoverage=on  Value=positioningmode
  Discrete-Time Integrator : DiscreteIntegrator  SampleTime=TimeStep  ICPrevOutput=DiscIntNeverNeededParam  ICPrevScaledInput=DiscIntNeverNeededParam
  Ground : Ground
  Ground1 : Ground
  Mux1 : Mux  Inputs=[3 3]
  Mux2 : Mux  Inputs=3
  Mux3 : Mux  Inputs=3
  Mux4 : Mux  Inputs=3
  Mux5 : Mux  Inputs=[3 3]
  Mux6 : Mux  Inputs=[6 3]
  Switch : Switch  Threshold=0.5
  Transformation_BODY2GLOBAL : PreScanSimulinkLibrary/Simple_Vehicle_Dynamics/Chassis/MuxDynState/Transformation_BODY2GLOBAL  SystemSampleTime=-1  Latency=0  AutoFrameSizeCalculation=off
  mux3 : Mux  Inputs=3
  state : Outport
  wires:
  Constant/1 -> Switch/2
  Mux6/1 -> state/1
  Mux4/1 -> Mux1/1
  Mux5/1 -> Switch/3
  Mux1/1 -> Switch/1
  Switch/1 -> Mux6/1  "PosVeh wrt  GLOB"
  P [rad]/1 -> Mux3/2
  R [rad]/1 -> Mux3/1
  dz [m/s]/1 -> Mux2/3
  dy [m/s]/1 -> Mux2/2
  dx [m/s]/1 -> Mux2/1
  z [m]/1 -> Mux4/3
  y [m]/1 -> Mux4/2
  x [m]/1 -> Mux4/1
  Ground1/1 -> mux3/2  "pitch"
  Y [rad]/1 -> mux3/3, Mux3/3  "yaw"
  Mux3/1 -> Mux6/2
  Transformation_BODY2GLOBAL/1 -> Discrete-Time Integrator/1, Mux5/2  "VelVEH wrt  GLOB"
  mux3/1 -> Transformation_BODY2GLOBAL/2
  Ground/1 -> mux3/1  "roll"
  Mux2/1 -> Mux1/2, Transformation_BODY2GLOBAL/1
  Discrete-Time Integrator/1 -> Mux5/1  "PosVEH wrt  GLOB"

== system EMPlanner_cs/Box_1/SELF_Demux/compas converter ==
  rotz [rad] : Inport
  cart2compas : Subsystem
  rad2deg : Gain  Gain=180/pi
  heading [deg] : Outport
  wires:
  rad2deg/1 -> cart2compas/1(Angle [deg])
  rotz [rad]/1 -> rad2deg/1
  cart2compas/1(heading [deg]) -> heading [deg]/1

== system EMPlanner_cs/Box_10/Dynamics_Empty/MuxState ==
  note: mode: Dynamics
  note: mode: Positioning
  note: mode: Dynamics
      | VelVEHICLE
      | wrt VEH
  note: AnglesVEHICLE
      | wrtGLOB
  note: For state mode 'Dynamic' positions
      | are not taken into account, as they
      | are computed by integrating velocity.
      | Click annotation for Help.
  x [m] : Inport  SampleTime=TimeStep
  y [m] : Inport  Port=2  SampleTime=TimeStep
  z [m] : Inport  Port=3  SampleTime=TimeStep
  dx [m/s] : Inport  Port=4  SampleTime=TimeStep
  dy [m/s] : Inport  Port=5  SampleTime=TimeStep
  dz [m/s] : Inport  Port=6  SampleTime=TimeStep
  R [rad] : Inport  Port=7  SampleTime=TimeStep
  P [rad] : Inport  Port=8  SampleTime=TimeStep
  Y [rad] : Inport  Port=9  SampleTime=TimeStep
  Constant : Constant  DisableCoverage=on  Value=positioningmode
  Discrete-Time Integrator : DiscreteIntegrator  SampleTime=TimeStep  ICPrevOutput=DiscIntNeverNeededParam  ICPrevScaledInput=DiscIntNeverNeededParam
  Ground : Ground
  Ground1 : Ground
  Mux1 : Mux  Inputs=[3 3]
  Mux2 : Mux  Inputs=3
  Mux3 : Mux  Inputs=3
  Mux4 : Mux  Inputs=3
  Mux5 : Mux  Inputs=[3 3]
  Mux6 : Mux  Inputs=[6 3]
  Switch : Switch  Threshold=0.5
  Transformation_BODY2GLOBAL : PreScanSimulinkLibrary/Simple_Vehicle_Dynamics/Chassis/MuxDynState/Transformation_BODY2GLOBAL  SystemSampleTime=-1  Latency=0  AutoFrameSizeCalculation=off
  mux3 : Mux  Inputs=3
  state : Outport
  wires:
  Constant/1 -> Switch/2
  Mux6/1 -> state/1
  Mux4/1 -> Mux1/1
  Mux5/1 -> Switch/3
  Mux1/1 -> Switch/1
  Switch/1 -> Mux6/1  "PosVeh wrt  GLOB"
  P [rad]/1 -> Mux3/2
  R [rad]/1 -> Mux3/1
  dz [m/s]/1 -> Mux2/3
  dy [m/s]/1 -> Mux2/2
  dx [m/s]/1 -> Mux2/1
  z [m]/1 -> Mux4/3
  y [m]/1 -> Mux4/2
  x [m]/1 -> Mux4/1
  Ground1/1 -> mux3/2  "pitch"
  Y [rad]/1 -> mux3/3, Mux3/3  "yaw"
  Mux3/1 -> Mux6/2
  Transformation_BODY2GLOBAL/1 -> Discrete-Time Integrator/1, Mux5/2  "VelVEH wrt  GLOB"
  mux3/1 -> Transformation_BODY2GLOBAL/2
  Ground/1 -> mux3/1  "roll"
  Mux2/1 -> Mux1/2, Transformation_BODY2GLOBAL/1
  Discrete-Time Integrator/1 -> Mux5/1  "PosVEH wrt  GLOB"

== system EMPlanner_cs/Box_10/SELF_Demux/compas converter ==
  rotz [rad] : Inport
  cart2compas : Subsystem
  rad2deg : Gain  Gain=180/pi
  heading [deg] : Outport
  wires:
  rad2deg/1 -> cart2compas/1(Angle [deg])
  rotz [rad]/1 -> rad2deg/1
  cart2compas/1(heading [deg]) -> heading [deg]/1

== system EMPlanner_cs/Box_11/Dynamics_Empty/MuxState ==
  note: mode: Dynamics
  note: mode: Positioning
  note: mode: Dynamics
      | VelVEHICLE
      | wrt VEH
  note: AnglesVEHICLE
      | wrtGLOB
  note: For state mode 'Dynamic' positions
      | are not taken into account, as they
      | are computed by integrating velocity.
      | Click annotation for Help.
  x [m] : Inport  SampleTime=TimeStep
  y [m] : Inport  Port=2  SampleTime=TimeStep
  z [m] : Inport  Port=3  SampleTime=TimeStep
  dx [m/s] : Inport  Port=4  SampleTime=TimeStep
  dy [m/s] : Inport  Port=5  SampleTime=TimeStep
  dz [m/s] : Inport  Port=6  SampleTime=TimeStep
  R [rad] : Inport  Port=7  SampleTime=TimeStep
  P [rad] : Inport  Port=8  SampleTime=TimeStep
  Y [rad] : Inport  Port=9  SampleTime=TimeStep
  Constant : Constant  DisableCoverage=on  Value=positioningmode
  Discrete-Time Integrator : DiscreteIntegrator  SampleTime=TimeStep  ICPrevOutput=DiscIntNeverNeededParam  ICPrevScaledInput=DiscIntNeverNeededParam
  Ground : Ground
  Ground1 : Ground
  Mux1 : Mux  Inputs=[3 3]
  Mux2 : Mux  Inputs=3
  Mux3 : Mux  Inputs=3
  Mux4 : Mux  Inputs=3
  Mux5 : Mux  Inputs=[3 3]
  Mux6 : Mux  Inputs=[6 3]
  Switch : Switch  Threshold=0.5
  Transformation_BODY2GLOBAL : PreScanSimulinkLibrary/Simple_Vehicle_Dynamics/Chassis/MuxDynState/Transformation_BODY2GLOBAL  SystemSampleTime=-1  Latency=0  AutoFrameSizeCalculation=off
  mux3 : Mux  Inputs=3
  state : Outport
  wires:
  Constant/1 -> Switch/2
  Mux6/1 -> state/1
  Mux4/1 -> Mux1/1
  Mux5/1 -> Switch/3
  Mux1/1 -> Switch/1
  Switch/1 -> Mux6/1  "PosVeh wrt  GLOB"
  P [rad]/1 -> Mux3/2
  R [rad]/1 -> Mux3/1
  dz [m/s]/1 -> Mux2/3
  dy [m/s]/1 -> Mux2/2
  dx [m/s]/1 -> Mux2/1
  z [m]/1 -> Mux4/3
  y [m]/1 -> Mux4/2
  x [m]/1 -> Mux4/1
  Ground1/1 -> mux3/2  "pitch"
  Y [rad]/1 -> mux3/3, Mux3/3  "yaw"
  Mux3/1 -> Mux6/2
  Transformation_BODY2GLOBAL/1 -> Discrete-Time Integrator/1, Mux5/2  "VelVEH wrt  GLOB"
  mux3/1 -> Transformation_BODY2GLOBAL/2
  Ground/1 -> mux3/1  "roll"
  Mux2/1 -> Mux1/2, Transformation_BODY2GLOBAL/1
  Discrete-Time Integrator/1 -> Mux5/1  "PosVEH wrt  GLOB"

== system EMPlanner_cs/Box_11/SELF_Demux/compas converter ==
  rotz [rad] : Inport
  cart2compas : Subsystem
  rad2deg : Gain  Gain=180/pi
  heading [deg] : Outport
  wires:
  rad2deg/1 -> cart2compas/1(Angle [deg])
  rotz [rad]/1 -> rad2deg/1
  cart2compas/1(heading [deg]) -> heading [deg]/1

== system EMPlanner_cs/Box_12/Dynamics_Empty/MuxState ==
  note: mode: Dynamics
  note: mode: Positioning
  note: mode: Dynamics
      | VelVEHICLE
      | wrt VEH
  note: AnglesVEHICLE
      | wrtGLOB
  note: For state mode 'Dynamic' positions
      | are not taken into account, as they
      | are computed by integrating velocity.
      | Click annotation for Help.
  x [m] : Inport  SampleTime=TimeStep
  y [m] : Inport  Port=2  SampleTime=TimeStep
  z [m] : Inport  Port=3  SampleTime=TimeStep
  dx [m/s] : Inport  Port=4  SampleTime=TimeStep
  dy [m/s] : Inport  Port=5  SampleTime=TimeStep
  dz [m/s] : Inport  Port=6  SampleTime=TimeStep
  R [rad] : Inport  Port=7  SampleTime=TimeStep
  P [rad] : Inport  Port=8  SampleTime=TimeStep
  Y [rad] : Inport  Port=9  SampleTime=TimeStep
  Constant : Constant  DisableCoverage=on  Value=positioningmode
  Discrete-Time Integrator : DiscreteIntegrator  SampleTime=TimeStep  ICPrevOutput=DiscIntNeverNeededParam  ICPrevScaledInput=DiscIntNeverNeededParam
  Ground : Ground
  Ground1 : Ground
  Mux1 : Mux  Inputs=[3 3]
  Mux2 : Mux  Inputs=3
  Mux3 : Mux  Inputs=3
  Mux4 : Mux  Inputs=3
  Mux5 : Mux  Inputs=[3 3]
  Mux6 : Mux  Inputs=[6 3]
  Switch : Switch  Threshold=0.5
  Transformation_BODY2GLOBAL : PreScanSimulinkLibrary/Simple_Vehicle_Dynamics/Chassis/MuxDynState/Transformation_BODY2GLOBAL  SystemSampleTime=-1  Latency=0  AutoFrameSizeCalculation=off
  mux3 : Mux  Inputs=3
  state : Outport
  wires:
  Constant/1 -> Switch/2
  Mux6/1 -> state/1
  Mux4/1 -> Mux1/1
  Mux5/1 -> Switch/3
  Mux1/1 -> Switch/1
  Switch/1 -> Mux6/1  "PosVeh wrt  GLOB"
  P [rad]/1 -> Mux3/2
  R [rad]/1 -> Mux3/1
  dz [m/s]/1 -> Mux2/3
  dy [m/s]/1 -> Mux2/2
  dx [m/s]/1 -> Mux2/1
  z [m]/1 -> Mux4/3
  y [m]/1 -> Mux4/2
  x [m]/1 -> Mux4/1
  Ground1/1 -> mux3/2  "pitch"
  Y [rad]/1 -> mux3/3, Mux3/3  "yaw"
  Mux3/1 -> Mux6/2
  Transformation_BODY2GLOBAL/1 -> Discrete-Time Integrator/1, Mux5/2  "VelVEH wrt  GLOB"
  mux3/1 -> Transformation_BODY2GLOBAL/2
  Ground/1 -> mux3/1  "roll"
  Mux2/1 -> Mux1/2, Transformation_BODY2GLOBAL/1
  Discrete-Time Integrator/1 -> Mux5/1  "PosVEH wrt  GLOB"

== system EMPlanner_cs/Box_12/SELF_Demux/compas converter ==
  rotz [rad] : Inport
  cart2compas : Subsystem
  rad2deg : Gain  Gain=180/pi
  heading [deg] : Outport
  wires:
  rad2deg/1 -> cart2compas/1(Angle [deg])
  rotz [rad]/1 -> rad2deg/1
  cart2compas/1(heading [deg]) -> heading [deg]/1

== system EMPlanner_cs/Box_2/Dynamics_Empty/MuxState ==
  note: mode: Dynamics
  note: mode: Positioning
  note: mode: Dynamics
      | VelVEHICLE
      | wrt VEH
  note: AnglesVEHICLE
      | wrtGLOB
  note: For state mode 'Dynamic' positions
      | are not taken into account, as they
      | are computed by integrating velocity.
      | Click annotation for Help.
  x [m] : Inport  SampleTime=TimeStep
  y [m] : Inport  Port=2  SampleTime=TimeStep
  z [m] : Inport  Port=3  SampleTime=TimeStep
  dx [m/s] : Inport  Port=4  SampleTime=TimeStep
  dy [m/s] : Inport  Port=5  SampleTime=TimeStep
  dz [m/s] : Inport  Port=6  SampleTime=TimeStep
  R [rad] : Inport  Port=7  SampleTime=TimeStep
  P [rad] : Inport  Port=8  SampleTime=TimeStep
  Y [rad] : Inport  Port=9  SampleTime=TimeStep
  Constant : Constant  DisableCoverage=on  Value=positioningmode
  Discrete-Time Integrator : DiscreteIntegrator  SampleTime=TimeStep  ICPrevOutput=DiscIntNeverNeededParam  ICPrevScaledInput=DiscIntNeverNeededParam
  Ground : Ground
  Ground1 : Ground
  Mux1 : Mux  Inputs=[3 3]
  Mux2 : Mux  Inputs=3
  Mux3 : Mux  Inputs=3
  Mux4 : Mux  Inputs=3
  Mux5 : Mux  Inputs=[3 3]
  Mux6 : Mux  Inputs=[6 3]
  Switch : Switch  Threshold=0.5
  Transformation_BODY2GLOBAL : PreScanSimulinkLibrary/Simple_Vehicle_Dynamics/Chassis/MuxDynState/Transformation_BODY2GLOBAL  SystemSampleTime=-1  Latency=0  AutoFrameSizeCalculation=off
  mux3 : Mux  Inputs=3
  state : Outport
  wires:
  Constant/1 -> Switch/2
  Mux6/1 -> state/1
  Mux4/1 -> Mux1/1
  Mux5/1 -> Switch/3
  Mux1/1 -> Switch/1
  Switch/1 -> Mux6/1  "PosVeh wrt  GLOB"
  P [rad]/1 -> Mux3/2
  R [rad]/1 -> Mux3/1
  dz [m/s]/1 -> Mux2/3
  dy [m/s]/1 -> Mux2/2
  dx [m/s]/1 -> Mux2/1
  z [m]/1 -> Mux4/3
  y [m]/1 -> Mux4/2
  x [m]/1 -> Mux4/1
  Ground1/1 -> mux3/2  "pitch"
  Y [rad]/1 -> mux3/3, Mux3/3  "yaw"
  Mux3/1 -> Mux6/2
  Transformation_BODY2GLOBAL/1 -> Discrete-Time Integrator/1, Mux5/2  "VelVEH wrt  GLOB"
  mux3/1 -> Transformation_BODY2GLOBAL/2
  Ground/1 -> mux3/1  "roll"
  Mux2/1 -> Mux1/2, Transformation_BODY2GLOBAL/1
  Discrete-Time Integrator/1 -> Mux5/1  "PosVEH wrt  GLOB"

== system EMPlanner_cs/Box_2/SELF_Demux/compas converter ==
  rotz [rad] : Inport
  cart2compas : Subsystem
  rad2deg : Gain  Gain=180/pi
  heading [deg] : Outport
  wires:
  rad2deg/1 -> cart2compas/1(Angle [deg])
  rotz [rad]/1 -> rad2deg/1
  cart2compas/1(heading [deg]) -> heading [deg]/1

== system EMPlanner_cs/Box_3/Dynamics_Empty/MuxState ==
  note: mode: Dynamics
  note: mode: Positioning
  note: mode: Dynamics
      | VelVEHICLE
      | wrt VEH
  note: AnglesVEHICLE
      | wrtGLOB
  note: For state mode 'Dynamic' positions
      | are not taken into account, as they
      | are computed by integrating velocity.
      | Click annotation for Help.
  x [m] : Inport  SampleTime=TimeStep
  y [m] : Inport  Port=2  SampleTime=TimeStep
  z [m] : Inport  Port=3  SampleTime=TimeStep
  dx [m/s] : Inport  Port=4  SampleTime=TimeStep
  dy [m/s] : Inport  Port=5  SampleTime=TimeStep
  dz [m/s] : Inport  Port=6  SampleTime=TimeStep
  R [rad] : Inport  Port=7  SampleTime=TimeStep
  P [rad] : Inport  Port=8  SampleTime=TimeStep
  Y [rad] : Inport  Port=9  SampleTime=TimeStep
  Constant : Constant  DisableCoverage=on  Value=positioningmode
  Discrete-Time Integrator : DiscreteIntegrator  SampleTime=TimeStep  ICPrevOutput=DiscIntNeverNeededParam  ICPrevScaledInput=DiscIntNeverNeededParam
  Ground : Ground
  Ground1 : Ground
  Mux1 : Mux  Inputs=[3 3]
  Mux2 : Mux  Inputs=3
  Mux3 : Mux  Inputs=3
  Mux4 : Mux  Inputs=3
  Mux5 : Mux  Inputs=[3 3]
  Mux6 : Mux  Inputs=[6 3]
  Switch : Switch  Threshold=0.5
  Transformation_BODY2GLOBAL : PreScanSimulinkLibrary/Simple_Vehicle_Dynamics/Chassis/MuxDynState/Transformation_BODY2GLOBAL  SystemSampleTime=-1  Latency=0  AutoFrameSizeCalculation=off
  mux3 : Mux  Inputs=3
  state : Outport
  wires:
  Constant/1 -> Switch/2
  Mux6/1 -> state/1
  Mux4/1 -> Mux1/1
  Mux5/1 -> Switch/3
  Mux1/1 -> Switch/1
  Switch/1 -> Mux6/1  "PosVeh wrt  GLOB"
  P [rad]/1 -> Mux3/2
  R [rad]/1 -> Mux3/1
  dz [m/s]/1 -> Mux2/3
  dy [m/s]/1 -> Mux2/2
  dx [m/s]/1 -> Mux2/1
  z [m]/1 -> Mux4/3
  y [m]/1 -> Mux4/2
  x [m]/1 -> Mux4/1
  Ground1/1 -> mux3/2  "pitch"
  Y [rad]/1 -> mux3/3, Mux3/3  "yaw"
  Mux3/1 -> Mux6/2
  Transformation_BODY2GLOBAL/1 -> Discrete-Time Integrator/1, Mux5/2  "VelVEH wrt  GLOB"
  mux3/1 -> Transformation_BODY2GLOBAL/2
  Ground/1 -> mux3/1  "roll"
  Mux2/1 -> Mux1/2, Transformation_BODY2GLOBAL/1
  Discrete-Time Integrator/1 -> Mux5/1  "PosVEH wrt  GLOB"

== system EMPlanner_cs/Box_3/SELF_Demux/compas converter ==
  rotz [rad] : Inport
  cart2compas : Subsystem
  rad2deg : Gain  Gain=180/pi
  heading [deg] : Outport
  wires:
  rad2deg/1 -> cart2compas/1(Angle [deg])
  rotz [rad]/1 -> rad2deg/1
  cart2compas/1(heading [deg]) -> heading [deg]/1

== system EMPlanner_cs/Box_4/Dynamics_Empty/MuxState ==
  note: mode: Dynamics
  note: mode: Positioning
  note: mode: Dynamics
      | VelVEHICLE
      | wrt VEH
  note: AnglesVEHICLE
      | wrtGLOB
  note: For state mode 'Dynamic' positions
      | are not taken into account, as they
      | are computed by integrating velocity.
      | Click annotation for Help.
  x [m] : Inport  SampleTime=TimeStep
  y [m] : Inport  Port=2  SampleTime=TimeStep
  z [m] : Inport  Port=3  SampleTime=TimeStep
  dx [m/s] : Inport  Port=4  SampleTime=TimeStep
  dy [m/s] : Inport  Port=5  SampleTime=TimeStep
  dz [m/s] : Inport  Port=6  SampleTime=TimeStep
  R [rad] : Inport  Port=7  SampleTime=TimeStep
  P [rad] : Inport  Port=8  SampleTime=TimeStep
  Y [rad] : Inport  Port=9  SampleTime=TimeStep
  Constant : Constant  DisableCoverage=on  Value=positioningmode
  Discrete-Time Integrator : DiscreteIntegrator  SampleTime=TimeStep  ICPrevOutput=DiscIntNeverNeededParam  ICPrevScaledInput=DiscIntNeverNeededParam
  Ground : Ground
  Ground1 : Ground
  Mux1 : Mux  Inputs=[3 3]
  Mux2 : Mux  Inputs=3
  Mux3 : Mux  Inputs=3
  Mux4 : Mux  Inputs=3
  Mux5 : Mux  Inputs=[3 3]
  Mux6 : Mux  Inputs=[6 3]
  Switch : Switch  Threshold=0.5
  Transformation_BODY2GLOBAL : PreScanSimulinkLibrary/Simple_Vehicle_Dynamics/Chassis/MuxDynState/Transformation_BODY2GLOBAL  SystemSampleTime=-1  Latency=0  AutoFrameSizeCalculation=off
  mux3 : Mux  Inputs=3
  state : Outport
  wires:
  Constant/1 -> Switch/2
  Mux6/1 -> state/1
  Mux4/1 -> Mux1/1
  Mux5/1 -> Switch/3
  Mux1/1 -> Switch/1
  Switch/1 -> Mux6/1  "PosVeh wrt  GLOB"
  P [rad]/1 -> Mux3/2
  R [rad]/1 -> Mux3/1
  dz [m/s]/1 -> Mux2/3
  dy [m/s]/1 -> Mux2/2
  dx [m/s]/1 -> Mux2/1
  z [m]/1 -> Mux4/3
  y [m]/1 -> Mux4/2
  x [m]/1 -> Mux4/1
  Ground1/1 -> mux3/2  "pitch"
  Y [rad]/1 -> mux3/3, Mux3/3  "yaw"
  Mux3/1 -> Mux6/2
  Transformation_BODY2GLOBAL/1 -> Discrete-Time Integrator/1, Mux5/2  "VelVEH wrt  GLOB"
  mux3/1 -> Transformation_BODY2GLOBAL/2
  Ground/1 -> mux3/1  "roll"
  Mux2/1 -> Mux1/2, Transformation_BODY2GLOBAL/1
  Discrete-Time Integrator/1 -> Mux5/1  "PosVEH wrt  GLOB"

== system EMPlanner_cs/Box_4/SELF_Demux/compas converter ==
  rotz [rad] : Inport
  cart2compas : Subsystem
  rad2deg : Gain  Gain=180/pi
  heading [deg] : Outport
  wires:
  rad2deg/1 -> cart2compas/1(Angle [deg])
  rotz [rad]/1 -> rad2deg/1
  cart2compas/1(heading [deg]) -> heading [deg]/1

== system EMPlanner_cs/Box_5/Dynamics_Empty/MuxState ==
  note: mode: Dynamics
  note: mode: Positioning
  note: mode: Dynamics
      | VelVEHICLE
      | wrt VEH
  note: AnglesVEHICLE
      | wrtGLOB
  note: For state mode 'Dynamic' positions
      | are not taken into account, as they
      | are computed by integrating velocity.
      | Click annotation for Help.
  x [m] : Inport  SampleTime=TimeStep
  y [m] : Inport  Port=2  SampleTime=TimeStep
  z [m] : Inport  Port=3  SampleTime=TimeStep
  dx [m/s] : Inport  Port=4  SampleTime=TimeStep
  dy [m/s] : Inport  Port=5  SampleTime=TimeStep
  dz [m/s] : Inport  Port=6  SampleTime=TimeStep
  R [rad] : Inport  Port=7  SampleTime=TimeStep
  P [rad] : Inport  Port=8  SampleTime=TimeStep
  Y [rad] : Inport  Port=9  SampleTime=TimeStep
  Constant : Constant  DisableCoverage=on  Value=positioningmode
  Discrete-Time Integrator : DiscreteIntegrator  SampleTime=TimeStep  ICPrevOutput=DiscIntNeverNeededParam  ICPrevScaledInput=DiscIntNeverNeededParam
  Ground : Ground
  Ground1 : Ground
  Mux1 : Mux  Inputs=[3 3]
  Mux2 : Mux  Inputs=3
  Mux3 : Mux  Inputs=3
  Mux4 : Mux  Inputs=3
  Mux5 : Mux  Inputs=[3 3]
  Mux6 : Mux  Inputs=[6 3]
  Switch : Switch  Threshold=0.5
  Transformation_BODY2GLOBAL : PreScanSimulinkLibrary/Simple_Vehicle_Dynamics/Chassis/MuxDynState/Transformation_BODY2GLOBAL  SystemSampleTime=-1  Latency=0  AutoFrameSizeCalculation=off
  mux3 : Mux  Inputs=3
  state : Outport
  wires:
  Constant/1 -> Switch/2
  Mux6/1 -> state/1
  Mux4/1 -> Mux1/1
  Mux5/1 -> Switch/3
  Mux1/1 -> Switch/1
  Switch/1 -> Mux6/1  "PosVeh wrt  GLOB"
  P [rad]/1 -> Mux3/2
  R [rad]/1 -> Mux3/1
  dz [m/s]/1 -> Mux2/3
  dy [m/s]/1 -> Mux2/2
  dx [m/s]/1 -> Mux2/1
  z [m]/1 -> Mux4/3
  y [m]/1 -> Mux4/2
  x [m]/1 -> Mux4/1
  Ground1/1 -> mux3/2  "pitch"
  Y [rad]/1 -> mux3/3, Mux3/3  "yaw"
  Mux3/1 -> Mux6/2
  Transformation_BODY2GLOBAL/1 -> Discrete-Time Integrator/1, Mux5/2  "VelVEH wrt  GLOB"
  mux3/1 -> Transformation_BODY2GLOBAL/2
  Ground/1 -> mux3/1  "roll"
  Mux2/1 -> Mux1/2, Transformation_BODY2GLOBAL/1
  Discrete-Time Integrator/1 -> Mux5/1  "PosVEH wrt  GLOB"

== system EMPlanner_cs/Box_5/SELF_Demux/compas converter ==
  rotz [rad] : Inport
  cart2compas : Subsystem
  rad2deg : Gain  Gain=180/pi
  heading [deg] : Outport
  wires:
  rad2deg/1 -> cart2compas/1(Angle [deg])
  rotz [rad]/1 -> rad2deg/1
  cart2compas/1(heading [deg]) -> heading [deg]/1
